simulink model "udp_test"  (R2021b)
settings: Solver=VariableStepAuto  StartTime=0.0  StopTime=inf  RelTol=1e-3
libraries: instrumentlib x2
settings Model: xpc_rtwmakecfg_data=_xpciplib__xpcetherlib__xpcether8255xlib__xpcetherGbElib__xpcnblib_  Creator=Barti  LastModifiedBy=adria
settings SolverCC: AlgebraicLoopSolver=TrustRegion
settings DataIOCC: ReturnWorkspaceOutputs=off
settings DebuggingCC: SFMachineParentedDataDiag=warning  ArithmeticOperatorsInVariantConditions=warning
settings SFSimCC: SimUseLocalCustomCode=off  CustomCodeUndefinedFunction=UseInterfaceOnly
settings RTWCC: RTWUseLocalCustomCode=off
settings CodeAppCC: StateflowObjectComments=on

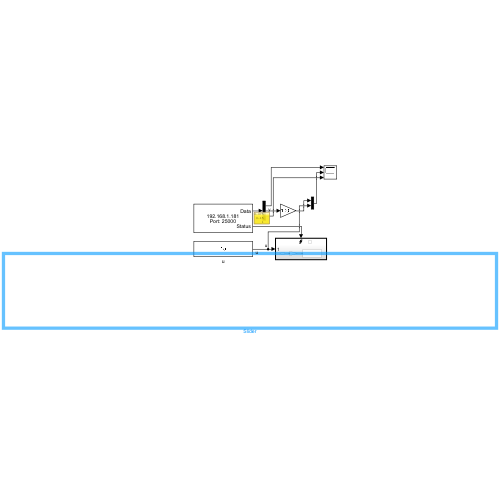
[thumbnail: Simulink's stored preview of the top-level diagram]
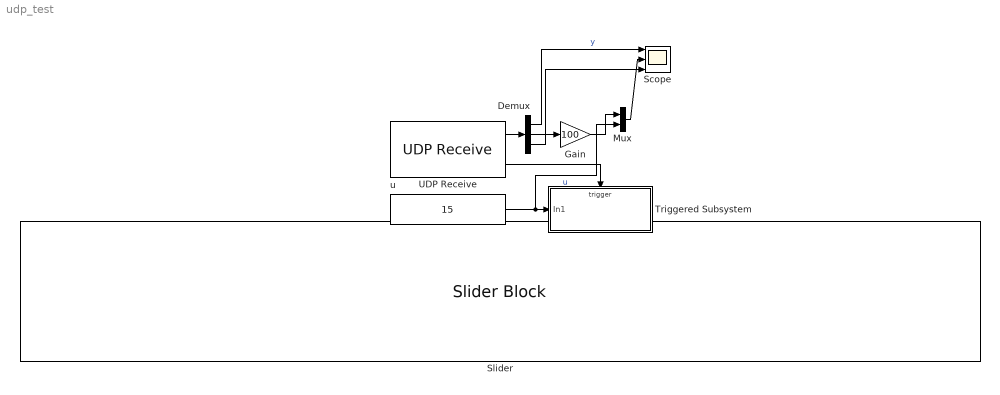
== system udp_test ==
  Demux : Demux  Outputs=3
  Gain : Gain  Gain=100
  Mux : Mux  Inputs=2
  Scope : Scope  NumInputPorts=3
  Slider : SliderBlock  LabelPosition=Hide  ScaleMin=-100  TickInterval=5
  Triggered Subsystem : Subsystem  TreatAsAtomicUnit=on
  UDP Receive : instrumentlib/UDP Receive  Host=192.168.1.248  Port=20001  LocalPort=25000  EnablePortSharing=off  GetLatestData=off  DataSize="[1  3]"  DataType=double  ASCIIFormatting=%d  Terminator=LF  ByteOrder=LittleEndian  EnableBlockingMode=off  Timeout=10  SampleTime=0.05  LocalAddress=192.168.1.181
  u : Constant  Value=15
  wires:
  UDP Receive/2 -> Triggered Subsystem/Trigger
  Demux/1 -> Scope/1  "y"
  UDP Receive/1 -> Demux/1
  u/1 -> Mux/2, Triggered Subsystem/1(In1)  "u"
  Mux/1 -> Scope/2
  Demux/3 -> Scope/3
  Demux/2 -> Gain/1
  Gain/1 -> Mux/1

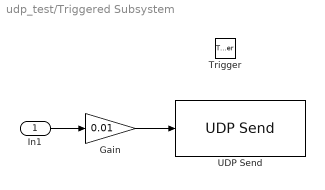
== system udp_test/Triggered Subsystem ==
  In1 : Inport
  Trigger : TriggerPort  VariantControl=(inherit)
  Gain : Gain  Gain=0.01
  UDP Send : instrumentlib/UDP Send  Host=192.168.1.248  Port=20002  LocalPort=25001  EnablePortSharing=off  ByteOrder=LittleEndian  OutputDatagramPacketSize=512  EnableBlockingMode=off  LocalAddress=192.168.1.181
  wires:
  In1/1 -> Gain/1
  Gain/1 -> UDP Send/1
